simulink model "ZNMDO"  (R2015a)
settings: Solver=ode45  StartTime=0.0  StopTime=500  RelTol=1e-3
libraries: simulink x9
settings Model: Creator=moham  LastModifiedBy=Ziad Ayman

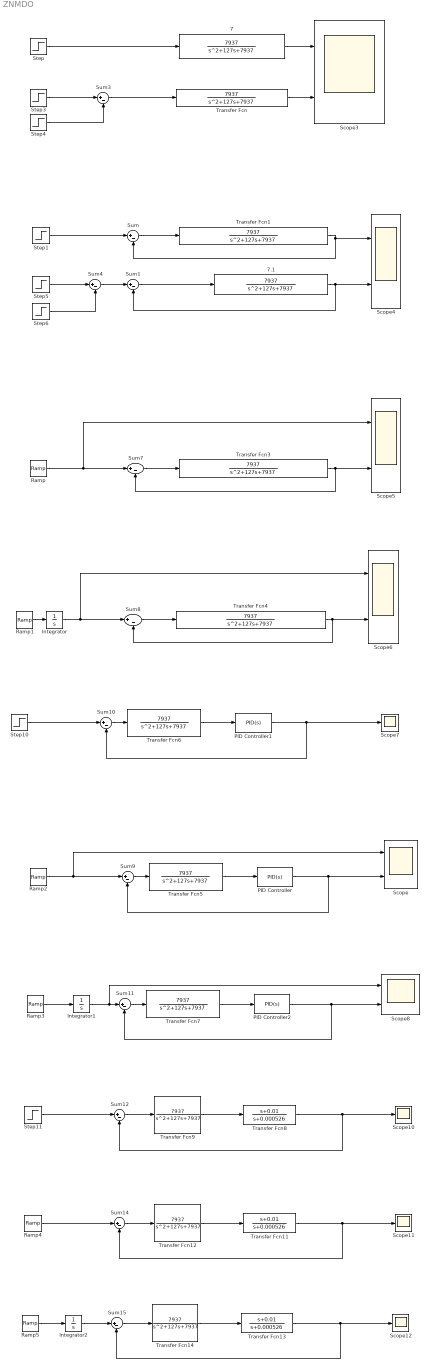
== system ZNMDO ==
  7 : TransferFcn  Numerator=[7937]  Denominator=[1 127 7937]
  7.1 : TransferFcn  Numerator=[7937]  Denominator=[1 127 7937]
  Integrator : Integrator
  Integrator1 : Integrator
  Integrator2 : Integrator
  PID Controller : simulink/Continuous/PID Controller  Controller=PID  TimeDomain=Continuous-time  SampleTime=-1  IntegratorMethod=Forward Euler  FilterMethod=Forward Euler  Form=Parallel  UseFilter=on  ControllerParametersSource=internal  P=0.1447  I=20  D=0.00126  N=1800  InitialConditionSource=internal  InitialConditionForIntegrator=0  InitialConditionForFilter=0  ExternalReset=none  LimitOutput=off  UpperSaturationLimit=inf  LowerSaturationLimit=-inf  LinearizeAsGain=on  AntiWindupMode=none  Kb=1  TrackingMode=off  Kt=1  PParamMin=[]  PParamMax=[]  IParamMin=[]  IParamMax=[]  DParamMin=[]  DParamMax=[]  NParamMin=[]  NParamMax=[]  KbParamMin=[]  KbParamMax=[]  KtParamMin=[]  KtParamMax=[]  POutMin=[]  POutMax=[]  IOutMin=[]  IOutMax=[]  DOutMin=[]  DOutMax=[]  NOutMin=[]  NOutMax=[]  KbOutMin=[]  KbOutMax=[]  KtOutMin=[]  KtOutMax=[]  IntegratorOutMin=[]  IntegratorOutMax=[]  FilterOutMin=[]  FilterOutMax=[]  SumOutMin=[]  SumOutMax=[]  SumI1OutMin=[]  SumI1OutMax=[]  SumI2OutMin=[]  SumI2OutMax=[]  SumI3OutMin=[]  SumI3OutMax=[]  SumDOutMin=[]  SumDOutMax=[]  SaturationOutMin=[]  SaturationOutMax=[]  IntegratorContinuousStateAttributes=''  IntegratorStateMustResolveToSignalObject=off  IntegratorRTWStateStorageClass=Auto  FilterContinuousStateAttributes=''  FilterStateMustResolveToSignalObject=off  FilterRTWStateStorageClass=Auto  DifferentiatorICPrevScaledInput=0  DifferentiatorOutMin=[]  DifferentiatorOutMax=[]
  PID Controller1 : simulink/Continuous/PID Controller  Controller=PID  TimeDomain=Continuous-time  SampleTime=-1  IntegratorMethod=Forward Euler  FilterMethod=Forward Euler  Form=Parallel  UseFilter=on  ControllerParametersSource=internal  P=0.1447  I=20  D=0.00126  N=1800  InitialConditionSource=internal  InitialConditionForIntegrator=0  InitialConditionForFilter=0  ExternalReset=none  LimitOutput=off  UpperSaturationLimit=inf  LowerSaturationLimit=-inf  LinearizeAsGain=on  AntiWindupMode=none  Kb=1  TrackingMode=off  Kt=1  PParamMin=[]  PParamMax=[]  IParamMin=[]  IParamMax=[]  DParamMin=[]  DParamMax=[]  NParamMin=[]  NParamMax=[]  KbParamMin=[]  KbParamMax=[]  KtParamMin=[]  KtParamMax=[]  POutMin=[]  POutMax=[]  IOutMin=[]  IOutMax=[]  DOutMin=[]  DOutMax=[]  NOutMin=[]  NOutMax=[]  KbOutMin=[]  KbOutMax=[]  KtOutMin=[]  KtOutMax=[]  IntegratorOutMin=[]  IntegratorOutMax=[]  FilterOutMin=[]  FilterOutMax=[]  SumOutMin=[]  SumOutMax=[]  SumI1OutMin=[]  SumI1OutMax=[]  SumI2OutMin=[]  SumI2OutMax=[]  SumI3OutMin=[]  SumI3OutMax=[]  SumDOutMin=[]  SumDOutMax=[]  SaturationOutMin=[]  SaturationOutMax=[]  IntegratorContinuousStateAttributes=''  IntegratorStateMustResolveToSignalObject=off  IntegratorRTWStateStorageClass=Auto  FilterContinuousStateAttributes=''  FilterStateMustResolveToSignalObject=off  FilterRTWStateStorageClass=Auto  DifferentiatorICPrevScaledInput=0  DifferentiatorOutMin=[]  DifferentiatorOutMax=[]
  PID Controller2 : simulink/Continuous/PID Controller  Controller=PID  TimeDomain=Continuous-time  SampleTime=-1  IntegratorMethod=Forward Euler  FilterMethod=Forward Euler  Form=Parallel  UseFilter=on  ControllerParametersSource=internal  P=0.1447  I=20  D=0.00126  N=1800  InitialConditionSource=internal  InitialConditionForIntegrator=0  InitialConditionForFilter=0  ExternalReset=none  LimitOutput=off  UpperSaturationLimit=inf  LowerSaturationLimit=-inf  LinearizeAsGain=on  AntiWindupMode=none  Kb=1  TrackingMode=off  Kt=1  PParamMin=[]  PParamMax=[]  IParamMin=[]  IParamMax=[]  DParamMin=[]  DParamMax=[]  NParamMin=[]  NParamMax=[]  KbParamMin=[]  KbParamMax=[]  KtParamMin=[]  KtParamMax=[]  POutMin=[]  POutMax=[]  IOutMin=[]  IOutMax=[]  DOutMin=[]  DOutMax=[]  NOutMin=[]  NOutMax=[]  KbOutMin=[]  KbOutMax=[]  KtOutMin=[]  KtOutMax=[]  IntegratorOutMin=[]  IntegratorOutMax=[]  FilterOutMin=[]  FilterOutMax=[]  SumOutMin=[]  SumOutMax=[]  SumI1OutMin=[]  SumI1OutMax=[]  SumI2OutMin=[]  SumI2OutMax=[]  SumI3OutMin=[]  SumI3OutMax=[]  SumDOutMin=[]  SumDOutMax=[]  SaturationOutMin=[]  SaturationOutMax=[]  IntegratorContinuousStateAttributes=''  IntegratorStateMustResolveToSignalObject=off  IntegratorRTWStateStorageClass=Auto  FilterContinuousStateAttributes=''  FilterStateMustResolveToSignalObject=off  FilterRTWStateStorageClass=Auto  DifferentiatorICPrevScaledInput=0  DifferentiatorOutMin=[]  DifferentiatorOutMax=[]
  Ramp{,1..5} (6 alike) : simulink/Sources/Ramp  slope=1  start=0  X0=0
  Scope{,3..6,8} (6 alike) : Scope  NumInputPorts=2
      Scope settings: YMin=-5~-5  YMax=5~5  SaveName=ScopeData6
      Scope3 settings: YMin=-5~-5  YMax=5~5  SaveName=ScopeData3
      Scope4 settings: YMin=-5~-5  YMax=5~5
      Scope5 settings: TimeRange=0.4999  YMin=0.5~0.2  YMax=1~0.5  SaveName=ScopeData4
      Scope6 settings: TimeRange=0.4999  YMin=0.5~0.2  YMax=1~0.5  SaveName=ScopeData5
      Scope8 settings: YMin=-5~-5  YMax=5~5  SaveName=ScopeData8
  Scope{7,10..12} (4 alike) : Scope
      Scope10 settings: SaveName=ScopeData9
      Scope11 settings: SaveName=ScopeData11
      Scope12 settings: SaveName=ScopeData12
      Scope7 settings: YMin=0  YMax=2  SaveName=ScopeData7
  Step : Step  Time=0  SampleTime=0.0001
  Step1 : Step  Time=0  SampleTime=0.0001
  Step10 : Step  Time=0  SampleTime=0
  Step11 : Step  Time=0  SampleTime=1
  Step3 : Step  Time=0  After=10000  SampleTime=0.0001
  Step4 : Step  Time=0.0000000000000001  After=10000  SampleTime=0.0001
  Step5 : Step  Time=0  After=10000  SampleTime=0.0001
  Step6 : Step  Time=0.0000000000000001  After=10000  SampleTime=0.0001
  Sum{,1,3..4,7..12,14..15} (12 alike) : Sum  Inputs=|+-
  Transfer Fcn{,1,3..7,9,12,14} (10 alike) : TransferFcn  Numerator=[7937]  Denominator=[1 127 7937]
  Transfer Fcn11 : TransferFcn  Numerator=[1 0.01]  Denominator=[1 0.000526]
  Transfer Fcn13 : TransferFcn  Numerator=[1 0.01]  Denominator=[1 0.000526]
  Transfer Fcn8 : TransferFcn  Numerator=[1 0.01]  Denominator=[1 0.000526]
  wires:
  Step/1 -> 7/1
  Step3/1 -> Sum3/1
  Step4/1 -> Sum3/2
  Sum3/1 -> Transfer Fcn/1
  7/1 -> Scope3/1
  Transfer Fcn/1 -> Scope3/2
  7.1/1 -> Scope4/2, Sum1/2
  Sum1/1 -> 7.1/1
  Step1/1 -> Sum/1
  Sum/1 -> Transfer Fcn1/1
  Transfer Fcn1/1 -> Scope4/1, Sum/2
  Step5/1 -> Sum4/1
  Step6/1 -> Sum4/2
  Sum4/1 -> Sum1/1
  Ramp/1 -> Sum7/1, Scope5/1
  Sum7/1 -> Transfer Fcn3/1
  Transfer Fcn3/1 -> Sum7/2, Scope5/2
  Ramp1/1 -> Integrator/1
  Sum8/1 -> Transfer Fcn4/1
  Transfer Fcn4/1 -> Sum8/2, Scope6/2
  Integrator/1 -> Sum8/1, Scope6/1
  Step10/1 -> Sum10/1
  Sum10/1 -> Transfer Fcn6/1
  PID Controller1/1 -> Sum10/2, Scope7/1
  Transfer Fcn6/1 -> PID Controller1/1
  Ramp2/1 -> Scope/1, Sum9/1
  Sum9/1 -> Transfer Fcn5/1
  PID Controller/1 -> Scope/2, Sum9/2
  Transfer Fcn5/1 -> PID Controller/1
  Ramp3/1 -> Integrator1/1
  Sum11/1 -> Transfer Fcn7/1
  PID Controller2/1 -> Sum11/2, Scope8/2
  Transfer Fcn7/1 -> PID Controller2/1
  Integrator1/1 -> Scope8/1, Sum11/1
  Step11/1 -> Sum12/1
  Transfer Fcn8/1 -> Sum12/2, Scope10/1
  Sum12/1 -> Transfer Fcn9/1
  Transfer Fcn9/1 -> Transfer Fcn8/1
  Ramp4/1 -> Sum14/1
  Transfer Fcn11/1 -> Sum14/2, Scope11/1
  Sum14/1 -> Transfer Fcn12/1
  Transfer Fcn12/1 -> Transfer Fcn11/1
  Ramp5/1 -> Integrator2/1
  Transfer Fcn13/1 -> Sum15/2, Scope12/1
  Sum15/1 -> Transfer Fcn14/1
  Transfer Fcn14/1 -> Transfer Fcn13/1
  Integrator2/1 -> Sum15/1
